simulink model "Assignment5"  (R2019a)
settings: Solver=FixedStepDiscrete  StartTime=0.0  StopTime=10  FixedStep=1  RelTol=1e-3
settings Model: Creator=balkr  LastModifiedBy=balkr

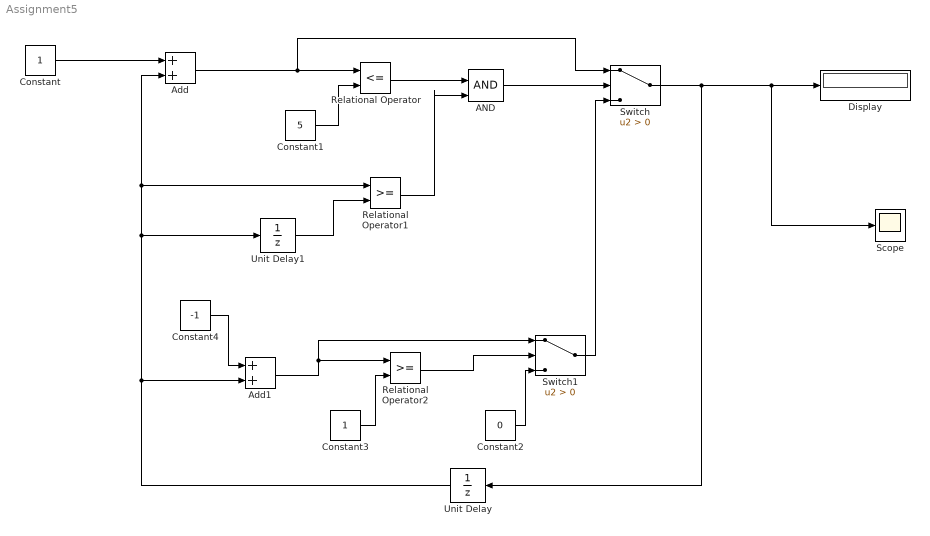
== system Assignment5 ==
  AND : Logic  IconShape=distinctive  AllPortsSameDT=off  OutDataTypeStr=boolean
  Add : Sum
  Add1 : Sum
  Constant : Constant
  Constant1 : Constant  Value=5
  Constant2 : Constant  Value=0
  Constant3 : Constant
  Constant4 : Constant  Value=-1
  Display : Display
  Relational Operator : RelationalOperator  Operator=<=  OutDataTypeStr=boolean  RndMeth=Simplest
  Relational Operator1 : RelationalOperator  OutDataTypeStr=boolean  RndMeth=Simplest
  Relational Operator2 : RelationalOperator  OutDataTypeStr=boolean  RndMeth=Simplest
  Scope : Scope
  Switch : Switch  Criteria=u2 > Threshold
  Switch1 : Switch  Criteria=u2 > Threshold
  Unit Delay : UnitDelay  InitialCondition=-1  SampleTime=-1  HasFrameUpgradeWarning=on
  Unit Delay1 : UnitDelay  InitialCondition=-1  SampleTime=-1  HasFrameUpgradeWarning=on
  wires:
  Constant3/1 -> Relational Operator2/2
  Add/1 -> Switch/1, Relational Operator/1
  Unit Delay/1 -> Add1/2, Unit Delay1/1, Relational Operator1/1, Add/2
  Switch/1 -> Unit Delay/1, Scope/1, Display/1
  Constant/1 -> Add/1
  Constant1/1 -> Relational Operator/2
  Constant2/1 -> Switch1/3
  Constant4/1 -> Add1/1
  Switch1/1 -> Switch/3
  Add1/1 -> Switch1/1, Relational Operator2/1
  AND/1 -> Switch/2
  Relational Operator1/1 -> AND/2
  Relational Operator2/1 -> Switch1/2
  Relational Operator/1 -> AND/1
  Unit Delay1/1 -> Relational Operator1/2
